simulink model "MSE452_Lab2_CHB_samplemodel_partC"  (R2023a)
settings: Solver=ode23t  StartTime=0.0  StopTime=0.1  MaxStep=1e-5  RelTol=1e-3  EnableMultiTasking=on
InitFcn:
  | ma=0.25
  | f1=60
  | T1=1/f1
  | fs_ps=720
  | Ts_ps=1/fs_ps
  | fs_ls=4320
  | Ts_ls=1/fs_ls
undefined symbols (not defined in the file): E
libraries: spsDCVoltageSourceLib x9, spsUniversalBridgeLib x9, simulink x9, spsTriangleGeneratorLib x9, spsVoltageMeasurementLib x5, spsSeriesRLCBranchLib x3, sps_lib x1
settings Model: Creator=jw  LastModifiedBy=mitch
settings SolverCC: AlgebraicLoopSolver=TrustRegion
settings DataIOCC: LimitDataPoints=on  SaveFormat=Array  SignalLoggingSaveFormat=ModelDataLogs  ReturnWorkspaceOutputs=off
settings OptimizationCC: InitFltsAndDblsToZero=on  LifeSpan=inf
settings DebuggingCC: SaveWithParameterizedLinksMsg=none  UnderspecifiedInitializationDetection=Classic  MergeDetectMultiDrivingBlocksExec=none  SignalResolutionControl=TryResolveAllWithWarning  SolverPrmCheckMsg=warning  MultiTaskDSMMsg=warning  MultiTaskCondExecSysMsg=none  FcnCallInpInsideContextMsg=warning  UnconnectedInputMsg=warning  UnconnectedOutputMsg=warning  UnconnectedLineMsg=warning  SFUnexpectedBacktrackingDiag=warning  SFNoUnconditionalDefaultTransitionDiag=warning  SFExecutionAtInitializationDiag=none  ArithmeticOperatorsInVariantConditions=warning
settings HardwareCC: ProdBitPerPointer=32  ProdBitPerSizeT=32  ProdBitPerPtrDiffT=32  ProdLargestAtomicFloat=None  ProdIntDivRoundTo=Undefined  ProdEndianess=Unspecified  ProdWordSize=32  ProdHWDeviceType=32-bit Generic
settings ModelReferenceCC: EnableRefExpFcnMdlSchedulingChecks=on  PropagateSignalLabelsOutOfModel=off
settings SFSimCC: CustomCodeUndefinedFunction=UseInterfaceOnly
settings CodeAppCC: StateflowObjectComments=on
settings GRTTargetCC: TargetFcnLib=ansi_tfl_tmw.mat  TargetLangStandard=C89/C90 (ANSI)  CombineOutputUpdateFcns=off  GRTInterface=on
settings ConfigComp: CovMetricSettings=dw  CovSaveCumulativeToWorkspaceVar=on  CovSaveSingleToWorkspaceVar=on

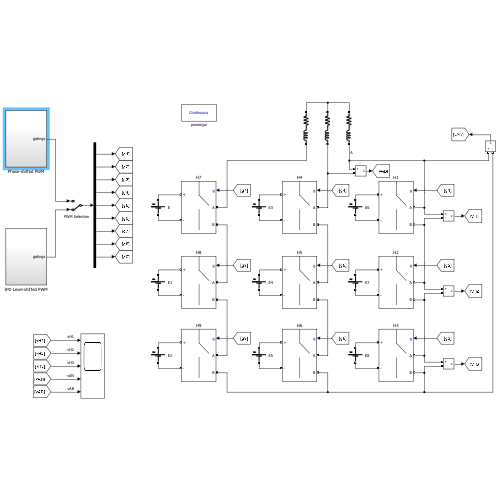
[thumbnail: Simulink's stored preview of the top-level diagram]
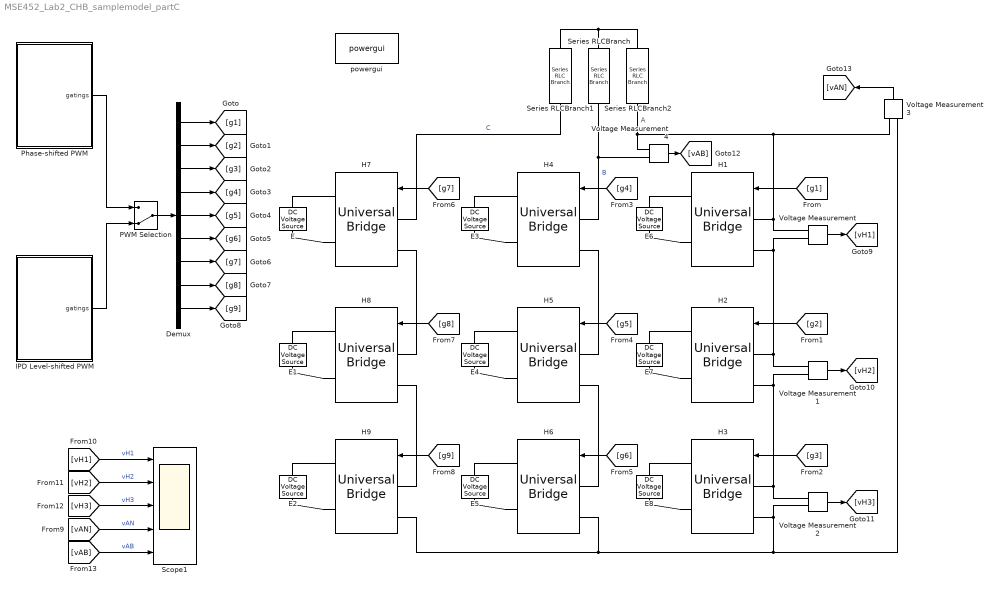
== system MSE452_Lab2_CHB_samplemodel_partC ==
  note: A
  Demux : Demux  Outputs=9
  E{,1..8} (9 alike) : spsDCVoltageSourceLib/DC Voltage Source  Amplitude=E  Measurements=None
  H{1..9} (9 alike) : spsUniversalBridgeLib/Universal Bridge  Arms=2  SnubberResistance=1e5  SnubberCapacitance=inf  Device=Ideal Switches  Ron=1e-3  Lon=0  ForwardVoltages="[  0  0  ]"  ForwardVoltage=0  GTOparameters=[ 10e-6 , 20e-6 ]  IGBTparameters=[ 1e-6 , 2e-6 ]  Measurements=None  Measurements_2=None  converterType=Rectifier
  IPD Level-shifted PWM : Subsystem
  PWM Selection : ManualSwitch  CurrentSetting=0
  Phase-shifted PWM : Subsystem
  Scope1 : Scope  NumInputPorts=5
  Series RLCBranch : spsSeriesRLCBranchLib/Series RLC Branch  LConnTagsString=__new0  RConnTagsString=__new0  BranchType=RL  Resistance=2.38  Inductance=3.05e-3  SetiL0=off  InitialCurrent=0  Capacitance=1e-6  Setx0=off  InitialVoltage=0  Measurements=None
  Series RLCBranch1 : spsSeriesRLCBranchLib/Series RLC Branch  LConnTagsString=__new0  RConnTagsString=__new0  BranchType=RL  Resistance=2.38  Inductance=3.05e-3  SetiL0=off  InitialCurrent=0  Capacitance=1e-6  Setx0=off  InitialVoltage=0  Measurements=None
  Series RLCBranch2 : spsSeriesRLCBranchLib/Series RLC Branch  LConnTagsString=__new0  RConnTagsString=__new0  BranchType=RL  Resistance=2.38  Inductance=3.05e-3  SetiL0=off  InitialCurrent=0  Capacitance=1e-6  Setx0=off  InitialVoltage=0  Measurements=None
  Voltage Measurement{,1..4} (5 alike) : spsVoltageMeasurementLib/Voltage Measurement  PhasorSimulation=off  OutputType=Complex  PSBequivalent=0
  powergui : sps_lib/powergui  Priority=1  SimulationMode=Continuous  SampleTime=50e-6  frequency=60  Iterations=50  frequencyindice=0  Pbase=100e6  ErrMax=1e-4  UnitsV=kV  UnitsW=MW  buscounter=0  FunctionMessages=off  echomessages=off  EnableUseOfTLC=off  CurrentSourceSwitches=off  DisableSnubberDevices=off  DisableRonSwitches=off  DisableVfSwitches=off  DisplayEquations=off  AutomaticDiscreteSolvers=off  SolverType=Tustin/Backward Euler (TBE)  Interpol=off  ExternalGateDelay=off  methode=off  Ts=100  x0status=blocks  SPID=on  SwTol=0  HookPort=off  NonlinearTolerance=1e-4  nMaxIteration=100  ContinueOnMaxIteration=off  RestoreLinks=warning  ResistiveCurrentMeasurement=off  Frange=[0:2:500]  Ylog=off  Xlog=on  ShowGrid=off  save=off  variable=ZData  structure=0  ZoomFFT=off  StartTime=0.0  cycles=1  DisplayStyle=1  fundamental=60  FreqAxis=off  MaxFrequency=1000  frequencyindicesteady=1  RmsSteady=1  display=off
  wires:
  [g1] -> H1/1
  [g2] -> H2/1
  [g3] -> H3/1
  [g4] -> H4/1
  [g5] -> H5/1
  [g6] -> H6/1
  [g7] -> H7/1
  [g8] -> H8/1
  [g9] -> H9/1
  Demux/1 -> [g1]
  Demux/2 -> [g2]
  Demux/3 -> [g3]
  Demux/4 -> [g4]
  Demux/5 -> [g5]
  Demux/6 -> [g6]
  Demux/7 -> [g7]
  Demux/8 -> [g8]
  Demux/9 -> [g9]
  Phase-shifted PWM/1(gatings) -> PWM Selection/1
  PWM Selection/1 -> Demux/1
  Voltage Measurement/1 -> [vH1]
  Voltage Measurement1/1 -> [vH2]
  Voltage Measurement2/1 -> [vH3]
  Voltage Measurement4/1 -> [vAB]
  Voltage Measurement3/1 -> [vAN]
  [vAN] -> Scope1/4  "vAN"
  [vH1] -> Scope1/1  "vH1"
  [vH2] -> Scope1/2  "vH2"
  [vH3] -> Scope1/3  "vH3"
  [vAB] -> Scope1/5  "vAB"
  IPD Level-shifted PWM/1(gatings) -> PWM Selection/2
  connections:
  H7/RConn2 -- E/LConn1
  E/RConn1 -- H7/RConn1
  E1/RConn1 -- H8/RConn1
  H8/RConn2 -- E1/LConn1
  E2/RConn1 -- H9/RConn1
  H9/RConn2 -- E2/LConn1
  H4/RConn2 -- E3/LConn1
  E5/RConn1 -- H6/RConn1
  E3/RConn1 -- H4/RConn1
  H6/RConn2 -- E5/LConn1
  E4/RConn1 -- H5/RConn1
  H5/RConn2 -- E4/LConn1
  H1/RConn2 -- E6/LConn1
  E8/RConn1 -- H3/RConn1
  E6/RConn1 -- H1/RConn1
  H3/RConn2 -- E8/LConn1
  E7/RConn1 -- H2/RConn1
  H2/RConn2 -- E7/LConn1
  H9/LConn2 -- H6/LConn2 -- H3/LConn2 -- Voltage Measurement2/LConn2 -- Voltage Measurement3/LConn2
  H9/LConn1 -- H8/LConn2
  H8/LConn1 -- H7/LConn2
  H4/LConn2 -- H5/LConn1
  H5/LConn2 -- H6/LConn1
  H1/LConn2 -- Voltage Measurement/LConn2 -- H2/LConn1 -- Voltage Measurement1/LConn1
  H2/LConn2 -- Voltage Measurement1/LConn2 -- H3/LConn1 -- Voltage Measurement2/LConn1
  H7/LConn1 -- Series RLCBranch1/RConn1  "C"
  Series RLCBranch/RConn1 -- H4/LConn1 -- Voltage Measurement4/LConn2  "B"
  H1/LConn1 -- Voltage Measurement/LConn1 -- Voltage Measurement3/LConn1 -- Series RLCBranch2/RConn1 -- Voltage Measurement4/LConn1
  Series RLCBranch1/LConn1 -- Series RLCBranch2/LConn1 -- Series RLCBranch/LConn1

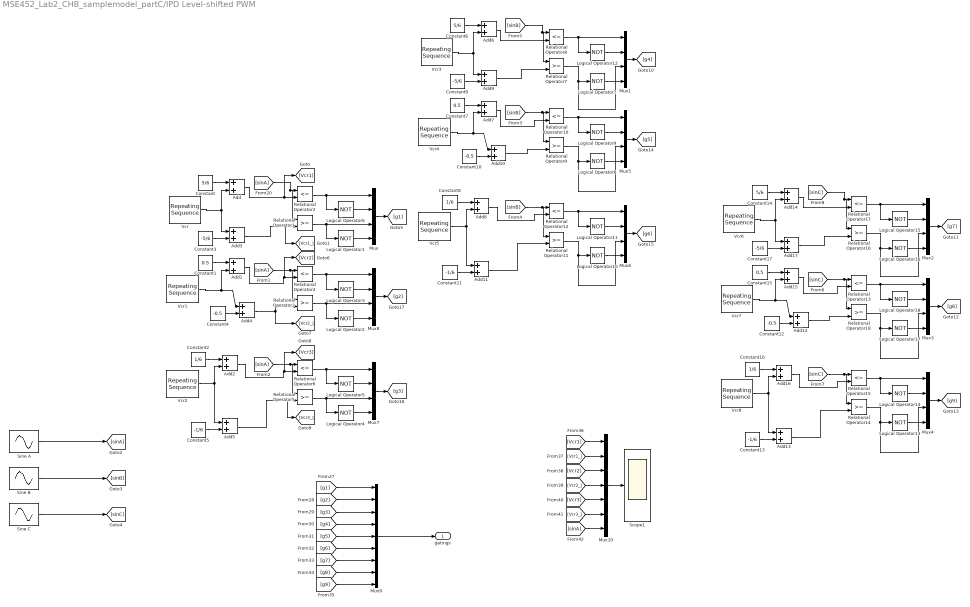
== system MSE452_Lab2_CHB_samplemodel_partC/IPD Level-shifted PWM ==
  Add{,1..17} (18 alike) : Sum
  Constant : Constant  Value=5/6
  Constant1 : Constant  Value=0.5
  Constant10 : Constant  Value=-0.5
  Constant11 : Constant  Value=-1/6
  Constant12 : Constant  Value=-0.5
  Constant13 : Constant  Value=-1/6
  Constant14 : Constant  Value=5/6
  Constant15 : Constant  Value=0.5
  Constant16 : Constant  Value=1/6
  Constant17 : Constant  Value=-5/6
  Constant2 : Constant  Value=1/6
  Constant3 : Constant  Value=-5/6
  Constant4 : Constant  Value=-0.5
  Constant5 : Constant  Value=-1/6
  Constant6 : Constant  Value=5/6
  Constant7 : Constant  Value=0.5
  Constant8 : Constant  Value=1/6
  Constant9 : Constant  Value=-5/6
  Logical Operator{1..18} (18 alike) : Logic  Operator=NOT  AllPortsSameDT=off  OutDataTypeStr=boolean
  Mux{,1..8} (9 alike) : Mux
  Mux10 : Mux  Inputs=7
  Mux9 : Mux  Inputs=9
  Relational Operator{1,3,5,7,9,11,14,16,18} (9 alike) : RelationalOperator  OutDataTypeStr=boolean  RndMeth=Simplest  InputSameDT=off
  Relational Operator{2,4,6,8,10,12..13,15,17} (9 alike) : RelationalOperator  Operator=<=  OutDataTypeStr=boolean  RndMeth=Simplest  InputSameDT=off
  Scope1 : Scope
  Sine A : Sin  Amplitude=ma  Frequency=2*pi*f1  SampleTime=0
  Sine B : Sin  Amplitude=ma  Frequency=2*pi*f1  Phase=-2/3*pi  SampleTime=0
  Sine C : Sin  Amplitude=ma  Frequency=2*pi*f1  Phase=2/3*pi  SampleTime=0
  Vcr{,1..8} (9 alike) : simulink/Sources/Repeating Sequence  rep_seq_t=[0 1/4*Ts_ls 3/4*Ts_ls Ts_ls]  rep_seq_y=[0 1/6 -1/6 0]
  gatings : Outport  VectorParamsAs1DForOutWhenUnconnected=off
  wires:
  Mux9/1 -> gatings/1
  Sine A/1 -> [sinA]
  Sine B/1 -> [sinB]
  Sine C/1 -> [sinC]
  Mux/1 -> [g1]
  Mux1/1 -> [g4]
  Mux2/1 -> [g7]
  Mux3/1 -> [g8]
  Mux4/1 -> [g9]
  Mux5/1 -> [g5]
  Mux6/1 -> [g6]
  Mux7/1 -> [g3]
  Mux8/1 -> [g2]
  [g1] -> Mux9/1
  [g2] -> Mux9/2
  [g3] -> Mux9/3
  [g4] -> Mux9/4
  [g5] -> Mux9/5
  [g6] -> Mux9/6
  [g7] -> Mux9/7
  [g8] -> Mux9/8
  [g9] -> Mux9/9
  [Vcr1] -> Mux10/1
  [Vcr1_] -> Mux10/2
  [Vcr2] -> Mux10/3
  [Vcr2_] -> Mux10/4
  [Vcr3] -> Mux10/5
  [Vcr3_] -> Mux10/6
  Mux10/1 -> Scope1/1
  [sinA] -> Mux10/7
  Relational Operator2/1 -> Mux/1, Logical Operator6/1
  Vcr/1 -> Add3/1, Add/2
  Relational Operator1/1 -> Mux/3, Logical Operator1/1
  Logical Operator6/1 -> Mux/2
  [sinA] -> Relational Operator1/1, Relational Operator2/1
  Logical Operator1/1 -> Mux/4
  Logical Operator2/1 -> Mux8/4
  [sinA] -> Relational Operator3/1, Relational Operator4/1
  Vcr1/1 -> Add4/1, Add1/2
  Logical Operator3/1 -> Mux8/2
  Relational Operator4/1 -> Mux8/1, Logical Operator3/1
  Relational Operator3/1 -> Logical Operator2/1, Mux8/3
  Relational Operator5/1 -> Logical Operator4/1, Mux7/3
  Relational Operator6/1 -> Mux7/1, Logical Operator5/1
  Logical Operator4/1 -> Mux7/4
  Logical Operator5/1 -> Mux7/2
  Vcr2/1 -> Add5/1, Add2/2
  [sinA] -> Relational Operator5/1, Relational Operator6/1
  Constant/1 -> Add/1
  Constant1/1 -> Add1/1
  Constant2/1 -> Add2/1
  Add1/1 -> [Vcr2], Relational Operator4/2
  Add/1 -> [Vcr1], Relational Operator2/2
  Add2/1 -> [Vcr3], Relational Operator6/2
  Constant3/1 -> Add3/2
  Add3/1 -> [Vcr1_], Relational Operator1/2
  Constant4/1 -> Add4/2
  Add4/1 -> Relational Operator3/2, [Vcr2_]
  Constant5/1 -> Add5/2
  Add5/1 -> [Vcr3_], Relational Operator5/2
  Relational Operator9/1 -> Mux5/3, Logical Operator8/1
  Relational Operator10/1 -> Mux5/1, Logical Operator9/1
  [sinB] -> Relational Operator11/1, Relational Operator12/1
  Logical Operator7/1 -> Mux1/4
  Relational Operator12/1 -> Mux6/1, Logical Operator11/1
  Logical Operator11/1 -> Mux6/2
  Logical Operator10/1 -> Mux6/4
  Constant7/1 -> Add7/1
  Logical Operator8/1 -> Mux5/4
  Add10/1 -> Relational Operator9/2
  Constant10/1 -> Add10/2
  Logical Operator9/1 -> Mux5/2
  Relational Operator11/1 -> Mux6/3, Logical Operator10/1
  Vcr4/1 -> Add10/1, Add7/2
  Add6/1 -> Relational Operator8/2
  Constant11/1 -> Add11/2
  Add9/1 -> Relational Operator7/2
  Vcr3/1 -> Add9/1, Add6/2
  Vcr5/1 -> Add11/1, Add8/2
  Constant6/1 -> Add6/1
  [sinB] -> Relational Operator9/1, Relational Operator10/1
  [sinB] -> Relational Operator7/1, Relational Operator8/1
  Logical Operator12/1 -> Mux1/2
  Relational Operator8/1 -> Mux1/1, Logical Operator12/1
  Relational Operator7/1 -> Mux1/3, Logical Operator7/1
  Add8/1 -> Relational Operator12/2
  Constant9/1 -> Add9/2
  Add11/1 -> Relational Operator11/2
  Add7/1 -> Relational Operator10/2
  Constant8/1 -> Add8/1
  Constant16/1 -> Add16/1
  Add17/1 -> Relational Operator16/2
  Add14/1 -> Relational Operator17/2
  Constant13/1 -> Add13/2
  Relational Operator16/1 -> Mux2/3, Logical Operator16/1
  Vcr6/1 -> Add17/1, Add14/2
  Relational Operator17/1 -> Mux2/1, Logical Operator15/1
  [sinC] -> Relational Operator16/1, Relational Operator17/1
  Relational Operator13/1 -> Mux3/1, Logical Operator18/1
  Relational Operator18/1 -> Mux3/3, Logical Operator17/1
  [sinC] -> Relational Operator18/1, Relational Operator13/1
  Relational Operator15/1 -> Mux4/1, Logical Operator14/1
  Add16/1 -> Relational Operator15/2
  Constant14/1 -> Add14/1
  Constant17/1 -> Add17/2
  Vcr8/1 -> Add13/1, Add16/2
  Logical Operator15/1 -> Mux2/2
  Logical Operator13/1 -> Mux4/4
  [sinC] -> Relational Operator14/1, Relational Operator15/1
  Logical Operator18/1 -> Mux3/2
  Add15/1 -> Relational Operator13/2
  Logical Operator14/1 -> Mux4/2
  Add13/1 -> Relational Operator14/2
  Logical Operator17/1 -> Mux3/4
  Relational Operator14/1 -> Mux4/3, Logical Operator13/1
  Constant15/1 -> Add15/1
  Vcr7/1 -> Add12/1, Add15/2
  Logical Operator16/1 -> Mux2/4
  Constant12/1 -> Add12/2
  Add12/1 -> Relational Operator18/2

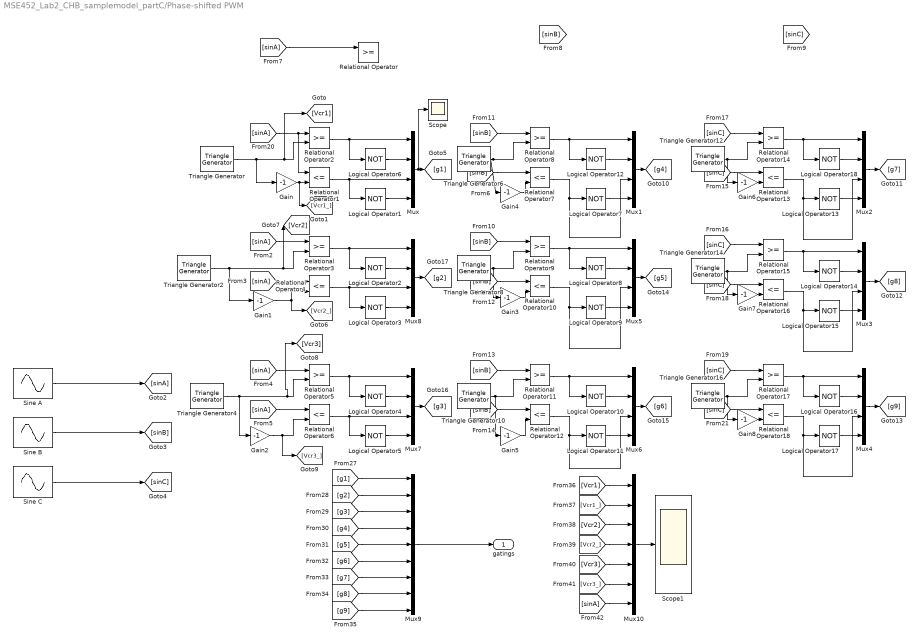
== system MSE452_Lab2_CHB_samplemodel_partC/Phase-shifted PWM ==
  Gain{,1..8} (9 alike) : Gain  Gain=-1
  Logical Operator{1..18} (18 alike) : Logic  Operator=NOT  AllPortsSameDT=off  OutDataTypeStr=boolean
  Mux{,1..8} (9 alike) : Mux
  Mux10 : Mux  Inputs=7
  Mux9 : Mux  Inputs=9
  Relational Operator{,2..3,5,8..9,11,14..15,17} (10 alike) : RelationalOperator  OutDataTypeStr=boolean  RndMeth=Simplest  InputSameDT=off
  Relational Operator{1,4,6..7,10,12..13,16,18} (9 alike) : RelationalOperator  Operator=<=  OutDataTypeStr=boolean  RndMeth=Simplest  InputSameDT=off
  Scope : Scope
  Scope1 : Scope
  Sine A : Sin  Amplitude=ma  Frequency=2*pi*f1  SampleTime=0
  Sine B : Sin  Amplitude=ma  Frequency=2*pi*f1  Phase=-2/3*pi  SampleTime=0
  Sine C : Sin  Amplitude=ma  Frequency=2*pi*f1  Phase=2/3*pi  SampleTime=0
  Triangle Generator : spsTriangleGeneratorLib/Triangle Generator  Freq=f2  Phase=0  Ts=0
  Triangle Generator10 : spsTriangleGeneratorLib/Triangle Generator  Freq=f2  Phase=120  Ts=0
  Triangle Generator12 : spsTriangleGeneratorLib/Triangle Generator  Freq=f2  Phase=0  Ts=0
  Triangle Generator14 : spsTriangleGeneratorLib/Triangle Generator  Freq=f2  Phase=60  Ts=0
  Triangle Generator16 : spsTriangleGeneratorLib/Triangle Generator  Freq=f2  Phase=120  Ts=0
  Triangle Generator2 : spsTriangleGeneratorLib/Triangle Generator  Freq=f2  Phase=60  Ts=0
  Triangle Generator4 : spsTriangleGeneratorLib/Triangle Generator  Freq=f2  Phase=120  Ts=0
  Triangle Generator6 : spsTriangleGeneratorLib/Triangle Generator  Freq=f2  Phase=0  Ts=0
  Triangle Generator8 : spsTriangleGeneratorLib/Triangle Generator  Freq=f2  Phase=60  Ts=0
  gatings : Outport  VectorParamsAs1DForOutWhenUnconnected=off
  wires:
  Mux9/1 -> gatings/1
  Sine A/1 -> [sinA]
  Sine B/1 -> [sinB]
  Sine C/1 -> [sinC]
  Mux/1 -> Scope/1, [g1]
  Mux1/1 -> [g4]
  Mux2/1 -> [g7]
  Mux3/1 -> [g8]
  Mux4/1 -> [g9]
  Mux5/1 -> [g5]
  Mux6/1 -> [g6]
  Mux7/1 -> [g3]
  Mux8/1 -> [g2]
  [g1] -> Mux9/1
  [g2] -> Mux9/2
  [g3] -> Mux9/3
  [g4] -> Mux9/4
  [g5] -> Mux9/5
  [g6] -> Mux9/6
  [g7] -> Mux9/7
  [g8] -> Mux9/8
  [g9] -> Mux9/9
  [Vcr1] -> Mux10/1
  [Vcr1_] -> Mux10/2
  [Vcr2] -> Mux10/3
  [Vcr2_] -> Mux10/4
  [Vcr3] -> Mux10/5
  [Vcr3_] -> Mux10/6
  Mux10/1 -> Scope1/1
  [sinA] -> Mux10/7
  [sinA] -> Relational Operator/1
  Logical Operator6/1 -> Mux/2
  Relational Operator2/1 -> Mux/1, Logical Operator6/1
  [sinA] -> Relational Operator1/1, Relational Operator2/1
  Triangle Generator/1 -> Gain/1, [Vcr1], Relational Operator2/2
  Relational Operator1/1 -> Mux/3, Logical Operator1/1
  Logical Operator1/1 -> Mux/4
  Relational Operator3/1 -> Mux8/1, Logical Operator2/1
  [sinA] -> Relational Operator3/1
  Triangle Generator2/1 -> Gain1/1, [Vcr2], Relational Operator3/2
  Logical Operator2/1 -> Mux8/2
  Relational Operator4/1 -> Mux8/3, Logical Operator3/1
  [sinA] -> Relational Operator4/1
  Logical Operator3/1 -> Mux8/4
  Relational Operator5/1 -> Mux7/1, Logical Operator4/1
  [sinA] -> Relational Operator5/1
  Triangle Generator4/1 -> Gain2/1, [Vcr3], Relational Operator5/2
  Logical Operator4/1 -> Mux7/2
  Relational Operator6/1 -> Mux7/3, Logical Operator5/1
  [sinA] -> Relational Operator6/1
  Gain2/1 -> [Vcr3_], Relational Operator6/2
  Logical Operator5/1 -> Mux7/4
  [sinB] -> Relational Operator10/1
  Relational Operator10/1 -> Mux5/3, Logical Operator9/1
  Logical Operator11/1 -> Mux6/4
  [sinB] -> Relational Operator7/1
  Triangle Generator10/1 -> Relational Operator11/2, Gain5/1
  Logical Operator10/1 -> Mux6/2
  Triangle Generator8/1 -> Relational Operator9/2, Gain3/1
  Relational Operator7/1 -> Mux1/3, Logical Operator7/1
  [sinB] -> Relational Operator9/1
  Logical Operator12/1 -> Mux1/2
  Relational Operator11/1 -> Mux6/1, Logical Operator10/1
  Logical Operator7/1 -> Mux1/4
  [sinB] -> Relational Operator8/1
  Relational Operator9/1 -> Mux5/1, Logical Operator8/1
  Relational Operator8/1 -> Mux1/1, Logical Operator12/1
  Logical Operator9/1 -> Mux5/4
  Relational Operator12/1 -> Mux6/3, Logical Operator11/1
  [sinB] -> Relational Operator11/1
  Logical Operator8/1 -> Mux5/2
  [sinB] -> Relational Operator12/1
  Triangle Generator6/1 -> Relational Operator8/2, Gain4/1
  [sinC] -> Relational Operator16/1
  Relational Operator16/1 -> Mux3/3, Logical Operator15/1
  Logical Operator17/1 -> Mux4/4
  [sinC] -> Relational Operator13/1
  Triangle Generator16/1 -> Relational Operator17/2, Gain8/1
  Logical Operator16/1 -> Mux4/2
  Triangle Generator14/1 -> Relational Operator15/2, Gain7/1
  Relational Operator13/1 -> Mux2/3, Logical Operator13/1
  [sinC] -> Relational Operator15/1
  Logical Operator18/1 -> Mux2/2
  Relational Operator17/1 -> Mux4/1, Logical Operator16/1
  Logical Operator13/1 -> Mux2/4
  [sinC] -> Relational Operator14/1
  Relational Operator15/1 -> Mux3/1, Logical Operator14/1
  Relational Operator14/1 -> Mux2/1, Logical Operator18/1
  Logical Operator15/1 -> Mux3/4
  Relational Operator18/1 -> Mux4/3, Logical Operator17/1
  [sinC] -> Relational Operator17/1
  Logical Operator14/1 -> Mux3/2
  [sinC] -> Relational Operator18/1
  Triangle Generator12/1 -> Relational Operator14/2, Gain6/1
  Gain/1 -> [Vcr1_], Relational Operator1/2
  Gain1/1 -> [Vcr2_], Relational Operator4/2
  Gain4/1 -> Relational Operator7/2
  Gain3/1 -> Relational Operator10/2
  Gain5/1 -> Relational Operator12/2
  Gain8/1 -> Relational Operator18/2
  Gain7/1 -> Relational Operator16/2
  Gain6/1 -> Relational Operator13/2
